simulink model "Questionno8"  (R2020a)
settings: Solver=VariableStepAuto  StartTime=0.0  StopTime=10.0  RelTol=1e-3
libraries: simulink x2
settings Model: Creator=anjal  LastModifiedBy=anjal

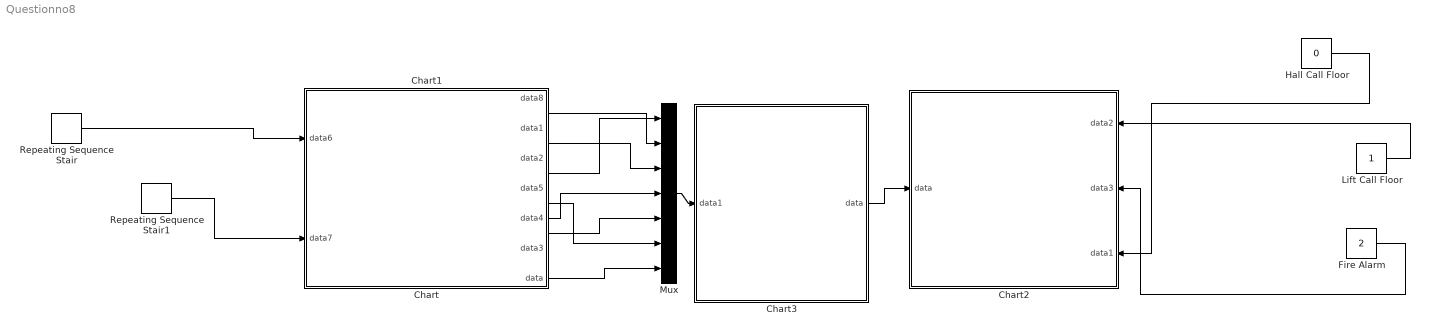
== system Questionno8 ==
  Chart : Stateflow chart  TreatAsAtomicUnit=on
  Chart1 : Stateflow chart  TreatAsAtomicUnit=on
      settings: PortSchema="{\"entries\":[{\"content\":{\"sides\":[{\"content\":{\"connectorIds\":[\"In2\",\"In3\"]},\"type\":\"ConnectorPlacement.EquallySpacedRectSide\",\"uuid\":\"67b6d9ef-859a-4c01-b832-abc99cd34797\"},{\"content\":{\"connectorIds\":[\"In1\",\"Out1\",\"Out2\",\"Out3\",\"Out4\",\"Out5\",\"Out6\"],\"side\":\"RIGHT\"},\"type\":\"ConnectorPlacement.EquallySpacedRectSide\",\"uuid\":\"083ee031-6bfc-4eb8-9ed5-c4f941c6653d\"},{\"content\":{\"connectorIds\":[],\"side\":\"TOP\"},\"type\":\"ConnectorPlacement.EquallySpacedRectSide\",\"uuid\":\"84dba6d3-d85b-4831-9ae6-a68157ba5486\"}]},\"type\":\"ConnectorPlacement.EquallySpacedConnector\",\"uuid\":\"38541822-6e4f-4e8f-9fff-49564061afb1\"}],\"packageUris\":[\"http://schema.mathworks.com/mf0/Connector/19700101\"],\"version\":\"1.0\"}"
  Chart2 : Stateflow chart  TreatAsAtomicUnit=on
      settings: PortSchema="{\"entries\":[{\"content\":{\"sides\":[{\"content\":{\"connectorIds\":[\"In4\"]},\"type\":\"ConnectorPlacement.EquallySpacedRectSide\",\"uuid\":\"9d12e941-f93e-4b81-ba54-9a45c14cbce8\"},{\"content\":{\"connectorIds\":[\"In1\",\"In2\",\"In3\"],\"side\":\"RIGHT\"},\"type\":\"ConnectorPlacement.EquallySpacedRectSide\",\"uuid\":\"45bb56a4-cc23-4366-923d-37100c39de85\"},{\"content\":{\"connectorIds\":[],\"side\":\"TOP\"},\"type\":\"ConnectorPlacement.EquallySpacedRectSide\",\"uuid\":\"f9aae596-f753-4979-aba1-1b0e4382f01c\"}]},\"type\":\"ConnectorPlacement.EquallySpacedConnector\",\"uuid\":\"93073253-c852-46b5-9272-3cf50cfecfd7\"}],\"packageUris\":[\"http://schema.mathworks.com/mf0/Connector/19700101\"],\"version\":\"1.0\"}"
  Chart3 : Stateflow chart  TreatAsAtomicUnit=on
  Fire Alarm : Constant  Value=2
  Hall Call Floor : Constant  Value=0
  Lift Call Floor : Constant
  Mux : Mux  Inputs=7
  Repeating Sequence Stair : simulink/Sources/Repeating Sequence Stair  OutValues=[3 1 4 2 1].'  tsamp=-1  OutMin=[]  OutMax=[]  OutDataTypeStr=double  OutputDataTypeScalingMode=double  OutDataType=fixdt(0,8)  ConRadixGroup=Best Precision: Vector-wise  OutScaling=2^-12
  Repeating Sequence Stair1 : simulink/Sources/Repeating Sequence Stair  OutValues=[3 1 4 2 1].'  tsamp=-1  OutMin=[]  OutMax=[]  OutDataTypeStr=double  OutputDataTypeScalingMode=double  OutDataType=fixdt(0,8)  ConRadixGroup=Best Precision: Vector-wise  OutScaling=2^-12
  wires:
  Chart/1(data1) -> Mux/2
  Chart/2(data2) -> Mux/3
  Chart/5(data3) -> Mux/5
  Chart/4(data4) -> Mux/6
  Chart/3(data5) -> Mux/1
  Repeating Sequence Stair/1 -> Chart1/2(data6)
  Repeating Sequence Stair1/1 -> Chart1/3(data7)
  Chart1/4(data4) -> Mux/4
  Chart1/6(data) -> Mux/7
  Hall Call Floor/1 -> Chart2/3(data1)
  Lift Call Floor/1 -> Chart2/1(data2)
  Fire Alarm/1 -> Chart2/2(data3)
  Chart3/1(data) -> Chart2/4(data)
  Mux/1 -> Chart3/1(data1)

== stateflow chart Questionno8/Chart2 ==
  state LiftControl1
    du: updateLiftcontrol;
    state Normal
    state Upshift
      en: count = 0;
      du: count = count+1;
    state Downshift
      en: count = 0;
      du: count = count+1;
    (default) -> Normal
    Normal -> Upshift [order 1] : [v>v_liftup]
        | /{Lift.UP;}
    Normal -> Downshift [order 2] : [v<v_liftdown]
        | /{Lift.DOWN;}
    Downshift -> Normal : [count > 3]
    Upshift -> Normal : [count > 3]
  state LiftControl
    state Floor_2
      en: floor= 2;
    state Floor_4
      en: floor = 4;
    state Floor_5
      en: floor = 4;
    state Floor_3
      en: floor = 3;
    state Floor_1
      en: floor = 1;
    (default) -> Floor_1
    Floor_2 -> Floor_3 [order 1] : UP
    Floor_1 -> Floor_2 : UP
    Floor_3 -> Floor_4 [order 1] : UP
    Floor_4 -> Floor_5 [order 2]
    Floor_5 -> Floor_4
    Floor_2 -> Floor_1 [order 2] : DOWN
    Floor_3 -> Floor_2 [order 2] : DOWN
    Floor_4 -> Floor_3 [order 1] : DOWN
  (default) -> LiftControl1 [order 1] : Liftcall
  (default) -> LiftControl [order 2]
  data: data2 input; data3 input; data1 input; data input
  events: UP local FUNCTION_CALL_EVENT; DOWN local FUNCTION_CALL_EVENT

== stateflow chart Questionno8/Chart ==
  state Stopped
    state Stopped_and_Waiting
      state Initializing
        entry:Motor=false;BrakesOff=false;Doors=false;
        DestinedReached=False;CommndConsidered=false;
      state FixingDesignation
        LastDesignination=WantedDesination;
      state SettingDown
        entry:Up=false;
      state SettingUp
        entry:Up=true
      state CommandAccepted
        CommandConsidered=true;
      (default) -> Initializing [order 1] : [LiftCall&&~CommandConsidered]
      Initializing -> FixingDesignation
      FixingDesignation -> SettingDown [order 3]
      FixingDesignation -> SettingUp [order 1] : [CurretPosition<LastPosition]
      (default) -> CommandAccepted [order 2]
    state Stopping_at_destination
      state StoppingLift
        entry:Motor=False;BrakesOff=False;
      state ErrorState
        entry:Doors=false;
      state OpeningDoors
        entry:DesitinationReached=True;Doors=true;
      (default) -> StoppingLift
      StoppingLift -> OpeningDoors [order 1] : [CurrentPosition~=LastDestination]
      StoppingLift -> ErrorState [order 2]
    (default) -> Stopped_and_Waiting
    FixingDesignation -> Stopping_at_destination [order 2] : [CurrentPosition==LastDestination]
  state Moving
    state StartingMotor
      entry:Motor=true;BrakesOff=true;Doors=false;
    state MovingUp
      entry:CurrentPosition=CurrentPosition + 1
    state MovingDown
      entry:CurrentPosition = CurrentPosition-1;
    (default) -> StartingMotor
    MovingDown -> MovingDown : [CurrentPosirion>LastDestination]
    MovingUp -> MovingUp : [CurrentPosition<LastDestination]
    StartingMotor -> MovingUp [order 1] : [Up]
    StartingMotor -> MovingDown [order 2] : [~Up]
  (default) -> Stopped
  Moving -> Stopping_at_destination : [CurrentPosition==LastPosition]
  Stopped_and_Waiting -> Moving : [CommandConsidered]
  data: data1 output; data2 output; data5 output; data4 output; data3 output; data output

== stateflow chart Questionno8/Chart3 ==
  state Elevator
    state Indside_Elevator_A
      state Off
        entry:
        Lift=0;
        state noSwitch
        state carSwitch
        (default) -> Elevator.Indside_Elevator_A.Off.noSwitch
        Elevator.Indside_Elevator_A.Off.noSwitch -> Elevator.Indside_Elevator_A.Off.carSwitch : [after(3,tick)]
      state carOn
        entry:
        lift=1;
      state liftoff
        entry:
        lift=-1;
      (default) -> Off
      carOn -> Off : [car2 > (car3-dT)]
      liftoff -> Off : [car2< (car3+dT)]
      Elevator.Indside_Elevator_A.Off.carSwitch -> carOn [order 1] : [car < (car-dT)]
      Elevator.Indside_Elevator_A.Off.carSwitch -> liftoff [order 2] : [car > (car+dT)]
    state ElevatorOff
      entry:
      LiftEntry=0;
      state noSwitch
      state carSwitch
      (default) -> Elevator.ElevatorOff.noSwitch
      Elevator.ElevatorOff.noSwitch -> Elevator.ElevatorOff.carSwitch : [after(3,tick)]
    (default) -> Indside_Elevator_A
    Indside_Elevator_A -> ElevatorOff : [car == 0]
    Elevator.ElevatorOff.carSwitch -> Indside_Elevator_A : [car == 1]
  data: data output; data1 input

== stateflow chart Questionno8/Chart1 ==
  state Stopped
    state Stopped_and_Waiting
      state Initializing
        entry:Motor=false;BrakesOff=false;Doors=false;
        DestinedReached=False;CommndConsidered=false;
      state FixingDesignation
        LastDesignination=WantedDesination;
      state SettingDown
        entry:Up=false;
      state SettingUp
        entry:Up=true
      state CommandAccepted
        CommandConsidered=true;
      (default) -> Initializing [order 1] : [LiftCall&&~CommandConsidered]
      Initializing -> FixingDesignation
      FixingDesignation -> SettingDown [order 3]
      FixingDesignation -> SettingUp [order 1] : [CurretPosition<LastPosition]
      (default) -> CommandAccepted [order 2]
    state Stopping_at_destination
      state StoppingLift
        entry:Motor=False;BrakesOff=False;
      state ErrorState
        entry:Doors=false;
      state OpeningDoors
        entry:DesitinationReached=True;Doors=true;
      (default) -> StoppingLift
      StoppingLift -> OpeningDoors [order 1] : [CurrentPosition~=LastDestination]
      StoppingLift -> ErrorState [order 2]
    (default) -> Stopped_and_Waiting
    FixingDesignation -> Stopping_at_destination [order 2] : [CurrentPosition==LastDestination]
  state Moving
    state StartingMotor
      entry:Motor=true;BrakesOff=true;Doors=false;
    state MovingUp
      entry:CurrentPosition=CurrentPosition + 1
    state MovingDown
      entry:CurrentPosition = CurrentPosition-1;
    (default) -> StartingMotor
    MovingDown -> MovingDown : [CurrentPosirion>LastDestination]
    MovingUp -> MovingUp : [CurrentPosition<LastDestination]
    StartingMotor -> MovingUp [order 1] : [Up]
    StartingMotor -> MovingDown [order 2] : [~Up]
  (default) -> Stopped
  Moving -> Stopping_at_destination : [CurrentPosition==LastPosition]
  Stopped_and_Waiting -> Moving : [CommandConsidered]
  data: data8 input; data1 output; data2 output; data5 output; data4 output; data3 output; data output; data6 input; data7 input
